simulink model "Dc_Dc_boost"  (R2024b)
settings: Solver=VariableStepAuto  StartTime=0.0  StopTime=10.0  RelTol=1e-3
undefined symbols (not defined in the file): Ts
libraries: spsCurrentMeasurementLib x3, spsSeriesRLCBranchLib x3, spsVoltageMeasurementLib x2, spsDCVoltageSourceLib x1, spsDiodeLib x1, spsGroundLib x1, spsMeanLib x1, spsMosfetLib x1, spsPWMGeneratorDCDCLib x1, sps_lib x1
settings Model: Creator=David  LastModifiedBy=David

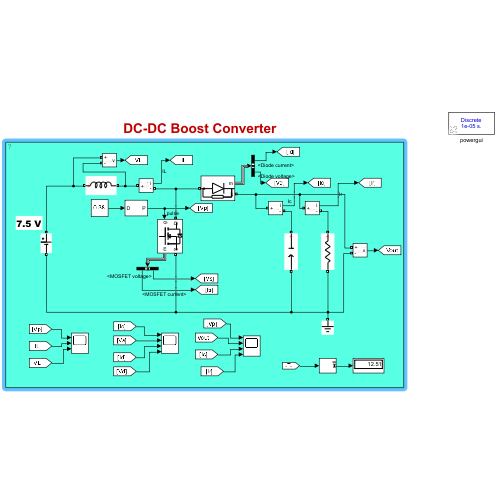
[thumbnail: Simulink's stored preview of the top-level diagram]
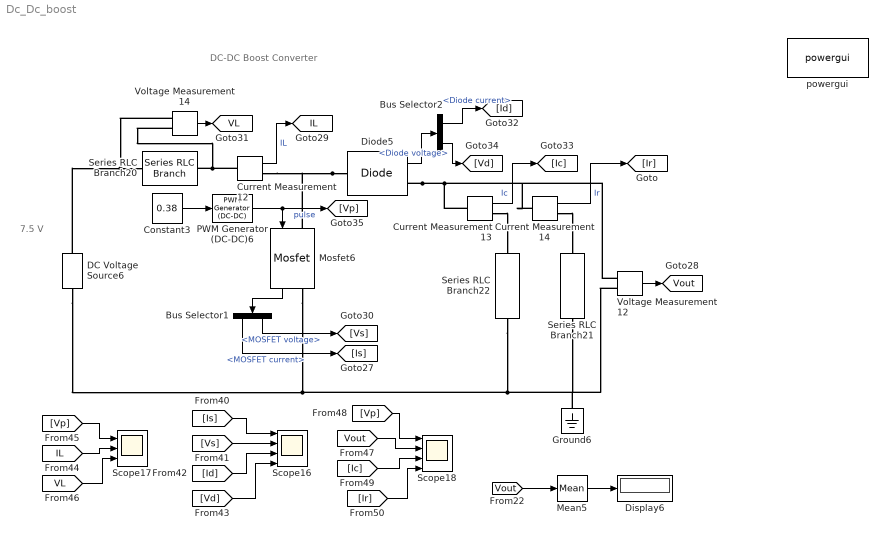
== system Dc_Dc_boost ==
  note: 7.5 V
  note: DC-DC Boost Converter
  Bus Selector1 : BusSelector  OutputSignals=MOSFET current,MOSFET voltage
  Bus Selector2 : BusSelector  OutputSignals=Diode current,Diode voltage
  Constant3 : Constant  Value=0.38
  Current Measurement12 : spsCurrentMeasurementLib/Current Measurement  PhasorSimulation=off  OutputType=Complex  PSBequivalent=0
  Current Measurement13 : spsCurrentMeasurementLib/Current Measurement  PhasorSimulation=off  OutputType=Complex  PSBequivalent=0
  Current Measurement14 : spsCurrentMeasurementLib/Current Measurement  PhasorSimulation=off  OutputType=Complex  PSBequivalent=0
  DC Voltage Source6 : spsDCVoltageSourceLib/DC Voltage Source  Amplitude=7.5  Measurements=None
  Diode5 : spsDiodeLib/Diode  Ron=1e-7  Lon=0  Vf=0  IC=0  UseSnubber=0  Rs=1e6  Cs=1e6  Measurements=on
  Display6 : Display
  Ground6 : spsGroundLib/Ground  LConnTagsString=a
  Mean5 : spsMeanLib/Mean  Freq=10000  Vinit=0  Ts=0
  Mosfet6 : spsMosfetLib/Mosfet  Ron=1e-7  Lon=0  Rd=1e-10  Vfd=0  IC=0  Rs=inf  Cs=0  Measurements=on
  PWM Generator (DC-DC)6 : spsPWMGeneratorDCDCLib/PWM Generator (DC-DC)  Fsw=10000  Ts=Ts
  Scope16 : Scope  NumInputPorts=4
  Scope17 : Scope  NumInputPorts=3
  Scope18 : Scope  NumInputPorts=4
  Series RLC Branch20 : spsSeriesRLCBranchLib/Series RLC Branch  LConnTagsString=__new0  RConnTagsString=__new0  BranchType=L  Resistance=0.000001  Inductance=0.0015  SetiL0=off  InitialCurrent=0  Capacitance=1e-6  Setx0=off  InitialVoltage=0  Measurements=None
  Series RLC Branch21 : spsSeriesRLCBranchLib/Series RLC Branch  LConnTagsString=__new0  RConnTagsString=__new0  BranchType=R  Resistance=12  Inductance=1e-3  SetiL0=off  InitialCurrent=0  Capacitance=1000e-6  Setx0=on  InitialVoltage=800  Measurements=None
  Series RLC Branch22 : spsSeriesRLCBranchLib/Series RLC Branch  LConnTagsString=__new0  RConnTagsString=__new0  BranchType=C  Resistance=6  Inductance=1e-3  SetiL0=off  InitialCurrent=0  Capacitance=416.67e-6  Setx0=off  InitialVoltage=800  Measurements=None
  Voltage Measurement12 : spsVoltageMeasurementLib/Voltage Measurement  PhasorSimulation=off  OutputType=Complex  PSBequivalent=0
  Voltage Measurement14 : spsVoltageMeasurementLib/Voltage Measurement  PhasorSimulation=off  OutputType=Complex  PSBequivalent=0
  powergui : sps_lib/powergui  Priority=1  SimulationMode=Discrete  SampleTime=Ts  frequency=60  Iterations=50  frequencyindice=0  Pbase=100e6  ErrMax=1e-4  UnitsV=kV  UnitsW=MW  buscounter=0  FunctionMessages=off  echomessages=off  EnableUseOfTLC=off  CurrentSourceSwitches=off  DisableSnubberDevices=off  DisableRonSwitches=off  DisableVfSwitches=off  DisplayEquations=off  AutomaticDiscreteSolvers=off  SolverType=Tustin/Backward Euler (TBE)  Interpol=off  ExternalGateDelay=off  methode=off  Ts=100  x0status=blocks  SPID=off  SwTol=0  HookPort=off  NonlinearTolerance=1e-4  nMaxIteration=100  ContinueOnMaxIteration=off  RestoreLinks=warning  ResistiveCurrentMeasurement=off  Frange=[0:2:500]  Ylog=off  Xlog=on  ShowGrid=off  save=off  variable=ZData  structure=0  ZoomFFT=off  StartTime=0.0  cycles=1  DisplayStyle=1  fundamental=60  FreqAxis=off  MaxFrequency=1000  frequencyindicesteady=1  RmsSteady=1  display=off
  tag scope: IL=global, VL=global, Vout=global
  wires:
  [Ir] -> Scope18/4
  [Vp] -> Scope17/1
  [Ic] -> Scope18/3
  Mean5/1 -> Display6/1
  Current Measurement14/1 -> [Ir]  "Ir"
  [Vout] -> Scope18/2
  Bus Selector2/2 -> [Vd]  "<Diode voltage>"
  Bus Selector1/1 -> [Is]  "<MOSFET current>"
  Current Measurement12/1 -> [IL]  "IL"
  Voltage Measurement12/1 -> [Vout]
  Mosfet6/1 -> Bus Selector1/1
  [Vout] -> Mean5/1
  [IL] -> Scope17/2
  Bus Selector2/1 -> [Id]  "<Diode current>"
  Constant3/1 -> PWM Generator (DC-DC)6/1
  [Vd] -> Scope16/4
  Diode5/1 -> Bus Selector2/1
  Current Measurement13/1 -> [Ic]  "Ic"
  [Is] -> Scope16/1
  [Vp] -> Scope18/1
  [Id] -> Scope16/3
  PWM Generator (DC-DC)6/1 -> [Vp], Mosfet6/1  "pulse"
  [VL] -> Scope17/3
  Bus Selector1/2 -> [Vs]  "<MOSFET voltage>"
  Voltage Measurement14/1 -> [VL]
  [Vs] -> Scope16/2
  connections:
  Mosfet6/RConn1 -- DC Voltage Source6/LConn1 -- Series RLC Branch22/RConn1 -- Ground6/LConn1 -- Voltage Measurement12/LConn2 -- Series RLC Branch21/RConn1
  Diode5/RConn1 -- Current Measurement13/LConn1 -- Current Measurement14/LConn1 -- Voltage Measurement12/LConn1
  Voltage Measurement14/LConn1 -- Series RLC Branch20/LConn1 -- DC Voltage Source6/RConn1
  Diode5/LConn1 -- Current Measurement12/RConn1 -- Mosfet6/LConn1
  Voltage Measurement14/LConn2 -- Series RLC Branch20/RConn1 -- Current Measurement12/LConn1
  Current Measurement13/RConn1 -- Series RLC Branch22/LConn1
  Current Measurement14/RConn1 -- Series RLC Branch21/LConn1
